simulink model "dx_hand_model"  (R2017b)
settings: Solver=ode3  StartTime=0.0  StopTime=inf  FixedStep=0.01  RelTol=1e-3  EnableMultiTasking=on
InitFcn:
  | cutFreq = 0.1; % T
  | sampleTime = 0.01;
  | filt = tf(1,[cutFreq 1]);
  | filt = c2d(filt,sampleTime);
  | 
  | cutFreq2 = 1;
  | filt2 = tf(1,[cutFreq2 1]);
  | filt2 = c2d(filt2,sampleTime);
  | 
  | cutFreq3 = 0.3;
  | filt3 = tf(1,[cutFreq3 1]);
  | filt3 = c2d(filt3,sampleTime);
  | 
  | update_param = 2;
  | 
  | ampliFactor = 1.60;
  | ampliFactorMiddle = 2.00;
  | ampliFactorDistal = 1;
  | 
  | % Set Hand Address
  | % RightHandAddress = '10.100.39.144';
  | RightHandAddress = '10.24.4.91';
  | Verosim = '10.100.39.22'
  | LeftHandAddress = '10.100.39.22'
  | 
  | max_force = 24; % Newton
model workspace (MAT data in the model file):
  SL_ROS_VariableLengthArrays_MaxSizes : struct (value not decoded)
libraries: robotlib x136, simulink_extras x27, simulink x16, etargetslib x2, dspnetwork x2
(part 3 of 19)

== system dx_hand_model/Get From Schunk/Get positions/Get Positions ==
  <Position> : Inport
  Data Type Conversion1 : DataTypeConversion  OutDataTypeStr=single
  Data Type Conversion2 : DataTypeConversion  OutDataTypeStr=single
  Demux : Demux  Outputs=9
  Display : Display
  Filter : Subsystem
  Filter1 : Subsystem
  Filter2 : Subsystem
  Filter3 : Subsystem
  Filter4 : Subsystem
  Filter5 : Subsystem
  Get Parameter3 : robotlib/Get Parameter  SourceLibraryInfo=This block requires Robotics System Toolbox  ParameterSource=Specify your own  ParameterName=/hand_exo/position/filt  ParameterType=double  ParameterMaxArrayLength=16  ParameterInitialValue=1.0  SampleTime=update_param  ShowErrorCodeOutput=on  ModelName=dx_hand_model  BlockId=ParamGet_dx_hand_model_3210
      settings: SourceProductName=Robotics System Toolbox  SourceProductBaseCode=RO
  Rate Transition : RateTransition
  Selector : Selector  IndexOptions=Index vector (dialog)  Indices=[1 2 3 4 5 6 7 8 9]  OutputSizes=1
  tag scope: act_IndexDistal=global, act_IndexProxi=global, act_MiddleDistal=global, act_MiddleProxi=global, act_Pinky=global, act_Ring=global
  wires:
  <Position>/1 -> Display/1, Selector/1
  Selector/1 -> Data Type Conversion2/1
  Demux/5 -> Filter2/2(in)
  Data Type Conversion2/1 -> Demux/1
  Demux/4 -> Filter1/2(in)
  Demux/6 -> Filter3/2(in)
  Filter1/1(out) -> [act_IndexProxi]
  Demux/3 -> Filter/2(in)
  Filter/1(out) -> [act_IndexDistal]
  Rate Transition/1 -> Data Type Conversion1/1
  Get Parameter3/1 -> Rate Transition/1
  Data Type Conversion1/1 -> Filter4/1(enable), Filter5/1(enable), Filter3/1(enable), Filter2/1(enable), Filter1/1(enable), Filter/1(enable)
  Filter2/1(out) -> [act_MiddleDistal]
  Filter3/1(out) -> [act_MiddleProxi]
  Filter5/1(out) -> [act_Ring]
  Demux/7 -> Filter5/2(in)
  Filter4/1(out) -> [act_Pinky]
  Demux/8 -> Filter4/2(in)

== system dx_hand_model/Index Finger/Force/Position Force Basic Architecture ==
  Display : Display
  Gain1 : Gain  Gain=1/360
  Maximum Torque : Gain  Gain=0.52
  Maximum Torque1 : Gain  Gain=0.04
  Mux : Mux  Inputs=2
  Normalize Current : Gain  Gain=1/688
  Sign : Gain  Gain=-1
  Sign1 : Gain
  pos_gains/dist : Subsystem
  pos_gains/prox : Subsystem
  force_vec : Outport
  wires:
  Mux/1 -> Display/1, force_vec/1
  pos_gains/dist/1(post_dist) -> Mux/2
  [CurrentIndexProximal] -> Normalize Current/1
  pos_gains/prox/1(post_prox) -> Mux/1
  [CurrentIndexDistal] -> Gain1/1
  Normalize Current/1 -> Maximum Torque/1
  Gain1/1 -> Maximum Torque1/1
  Maximum Torque/1 -> Sign/1
  Sign/1 -> pos_gains/prox/1(pre_prox)
  Maximum Torque1/1 -> Sign1/1
  Sign1/1 -> pos_gains/dist/1(pre_dist)

== system dx_hand_model/Index Finger/Force/Subsystem ==
  optim : Inport
  classic : Inport  Port=2
  Data Type Conversion1 : DataTypeConversion  OutDataTypeStr=single
  Get Parameter3 : robotlib/Get Parameter  SourceLibraryInfo=This block requires Robotics System Toolbox  ParameterSource=Specify your own  ParameterName=/hand_exo/index/modes/jacobian  ParameterType=double  ParameterMaxArrayLength=16  ParameterInitialValue=-1.0  SampleTime=update_param  ShowErrorCodeOutput=on  ModelName=dx_hand_model  BlockId=ParamGet_dx_hand_model_2644
      settings: SourceProductName=Robotics System Toolbox  SourceProductBaseCode=RO
  Rate Transition : RateTransition
  Switch : Switch  Criteria=u2 > Threshold
  J_out : Outport
  wires:
  Get Parameter3/1 -> Rate Transition/1
  Data Type Conversion1/1 -> Switch/2
  optim/1 -> Switch/1
  classic/1 -> Switch/3
  Switch/1 -> J_out/1
  Rate Transition/1 -> Data Type Conversion1/1

== system dx_hand_model/Index Finger/Pose Generator/Angular Potentiometer ==
  ADC : Inport
  Constant4 : Constant  Value=pi/2  OutDataTypeStr=single
  Data Type Conversion1 : DataTypeConversion  OutDataTypeStr=single
  Data Type Conversion2 : DataTypeConversion  OutDataTypeStr=double
  Display2 : Display
  Gain Aggiustato1 : Gain  Gain=330*pi/(1024*180)
  Get Parameter3 : robotlib/Get Parameter  SourceLibraryInfo=This block requires Robotics System Toolbox  ParameterSource=Specify your own  ParameterName=/hand_exo/index/calibration/set  ParameterType=double  ParameterMaxArrayLength=16  ParameterInitialValue=483  SampleTime=update_param  ShowErrorCodeOutput=on  ModelName=dx_hand_model  BlockId=ParamGet_dx_hand_model_2632
      settings: SourceProductName=Robotics System Toolbox  SourceProductBaseCode=RO
  Radians to Degrees1 : simulink_extras/Transformations/Radians to Degrees
  Rate Transition : RateTransition
  Set Parameter : robotlib/Set Parameter  SourceLibraryInfo=This block requires Robotics System Toolbox  ParameterSource=Specify your own  ParameterName=/hand_exo/index/calibration/get  ParameterType=double  ModelName=dx_hand_model  BlockId=ParamSet_dx_hand_model_2630
      settings: SourceProductName=Robotics System Toolbox  SourceProductBaseCode=RO
  Sum3 : Sum  Inputs=|+-
  Sum4 : Sum  Inputs=|+-
  Deg : Outport
  Rad : Outport  Port=2
  wires:
  Radians to Degrees1/1 -> Deg/1
  Sum4/1 -> Rad/1, Radians to Degrees1/1
  ADC/1 -> Data Type Conversion2/1, Sum3/1
  Sum3/1 -> Gain Aggiustato1/1
  Constant4/1 -> Sum4/1
  Gain Aggiustato1/1 -> Sum4/2
  Data Type Conversion2/1 -> Display2/1, Set Parameter/1
  Rate Transition/1 -> Data Type Conversion1/1
  Get Parameter3/1 -> Rate Transition/1
  Data Type Conversion1/1 -> Sum3/2

== system dx_hand_model/Index Finger/Pose Generator/Parameters ==
  In1 : Inport
  Data Type Conversion1 : DataTypeConversion  OutDataTypeStr=single
  Index Parameters : MATLAB Function  TreatAsAtomicUnit=on
  "to_dir_kin " : Outport
  wires:
  Index Parameters/1(y) -> Data Type Conversion1/1
  In1/1 -> Index Parameters/1(x)
  Data Type Conversion1/1 -> "to_dir_kin "/1

== system dx_hand_model/Index Finger/Pose Generator/Parametri Dito ==
  Get_from_ROS_param : Subsystem
  Hand Written : Subsystem
  Manual Switch : ManualSwitch
  Par : Outport
  wires:
  Get_from_ROS_param/1(param) -> Manual Switch/1
  Hand Written/1(param) -> Manual Switch/2
  Manual Switch/1 -> Par/1

== system dx_hand_model/Index Finger/Pose Generator/Record ==
  input : Inport
  param : Inport  Port=2
  output : Inport  Port=3
  Enable : EnablePort
  Mux2 : Mux  Inputs=3
  To Workspace : ToWorkspace  VariableName=index_pose  SampleTime=-1
  wires:
  Mux2/1 -> To Workspace/1
  param/1 -> Mux2/2
  output/1 -> Mux2/3
  input/1 -> Mux2/1

== system dx_hand_model/Index Finger/Pose Generator/Subsystem ==
  ADC : Inport
  Gain Aggiustato : Gain  Gain=50/1024
  "lx " : Outport
  wires:
  ADC/1 -> Gain Aggiustato/1
  Gain Aggiustato/1 -> "lx "/1

== system dx_hand_model/Index Finger/Position/Pre-Proc ==
  yes : Inport
  no : Inport  Port=2
  Data Type Conversion1 : DataTypeConversion  OutDataTypeStr=single
  Get Parameter3 : robotlib/Get Parameter  SourceLibraryInfo=This block requires Robotics System Toolbox  ParameterSource=Specify your own  ParameterName=/hand_exo/index/position/optim  ParameterType=double  ParameterMaxArrayLength=16  ParameterInitialValue=1.0  SampleTime=update_param  ShowErrorCodeOutput=on  ModelName=dx_hand_model  BlockId=ParamGet_dx_hand_model_3323
      settings: SourceProductName=Robotics System Toolbox  SourceProductBaseCode=RO
  Rate Transition : RateTransition
  Switch : Switch  Criteria=u2 > Threshold
  out : Outport
  wires:
  Get Parameter3/1 -> Rate Transition/1
  Rate Transition/1 -> Data Type Conversion1/1
  Data Type Conversion1/1 -> Switch/2
  yes/1 -> Switch/1
  no/1 -> Switch/3
  Switch/1 -> out/1

== system dx_hand_model/Index Finger/Position/active ==
  in : Inport
  Constant : Constant  Value=0  OutDataTypeStr=single
  Data Type Conversion1 : DataTypeConversion  OutDataTypeStr=single
  Get Parameter3 : robotlib/Get Parameter  SourceLibraryInfo=This block requires Robotics System Toolbox  ParameterSource=Specify your own  ParameterName=/hand_exo/index/position/proxi_d_act  ParameterType=double  ParameterMaxArrayLength=16  ParameterInitialValue=-1.0  SampleTime=update_param  ShowErrorCodeOutput=off  ModelName=dx_hand_model  BlockId=ParamGet_dx_hand_model_3464
      settings: SourceProductName=Robotics System Toolbox  SourceProductBaseCode=RO
  Rate Transition : RateTransition
  Switch : Switch  Criteria=u2 > Threshold
  out : Outport
  wires:
  Switch/1 -> out/1
  Data Type Conversion1/1 -> Switch/2
  Rate Transition/1 -> Data Type Conversion1/1
  Get Parameter3/1 -> Rate Transition/1
  in/1 -> Switch/1
  Constant/1 -> Switch/3

== system dx_hand_model/Index Finger/Position/active1 ==
  in : Inport
  Constant : Constant  Value=0  OutDataTypeStr=single
  Data Type Conversion1 : DataTypeConversion  OutDataTypeStr=single
  Get Parameter3 : robotlib/Get Parameter  SourceLibraryInfo=This block requires Robotics System Toolbox  ParameterSource=Specify your own  ParameterName=/hand_exo/index/position/dist_d_act  ParameterType=double  ParameterMaxArrayLength=16  ParameterInitialValue=-1.0  SampleTime=update_param  ShowErrorCodeOutput=off  ModelName=dx_hand_model  BlockId=ParamGet_dx_hand_model_3474
      settings: SourceProductName=Robotics System Toolbox  SourceProductBaseCode=RO
  Rate Transition : RateTransition
  Switch : Switch  Criteria=u2 > Threshold
  out : Outport
  wires:
  Switch/1 -> out/1
  Data Type Conversion1/1 -> Switch/2
  Rate Transition/1 -> Data Type Conversion1/1
  Get Parameter3/1 -> Rate Transition/1
  in/1 -> Switch/1
  Constant/1 -> Switch/3

== system dx_hand_model/Index Finger/Position/setGain ==
  in : Inport
  Data Type Conversion1 : DataTypeConversion  OutDataTypeStr=single
  Get Parameter3 : robotlib/Get Parameter  SourceLibraryInfo=This block requires Robotics System Toolbox  ParameterSource=Specify your own  ParameterName=/hand_exo/index/position/kp_p  ParameterType=double  ParameterMaxArrayLength=16  ParameterInitialValue=1.2  SampleTime=update_param  ShowErrorCodeOutput=off  ModelName=dx_hand_model  BlockId=ParamGet_dx_hand_model_3283
      settings: SourceProductName=Robotics System Toolbox  SourceProductBaseCode=RO
  Product : Product
  Rate Transition : RateTransition
  out : Outport
  wires:
  Product/1 -> out/1
  Data Type Conversion1/1 -> Product/1
  in/1 -> Product/2
  Rate Transition/1 -> Data Type Conversion1/1
  Get Parameter3/1 -> Rate Transition/1

== system dx_hand_model/Index Finger/Position/setGain  ==
  in : Inport
  Data Type Conversion1 : DataTypeConversion  OutDataTypeStr=single
  Get Parameter3 : robotlib/Get Parameter  SourceLibraryInfo=This block requires Robotics System Toolbox  ParameterSource=Specify your own  ParameterName=/hand_exo/index/position/kp_d  ParameterType=double  ParameterMaxArrayLength=16  ParameterInitialValue=0.2  SampleTime=update_param  ShowErrorCodeOutput=off  ModelName=dx_hand_model  BlockId=ParamGet_dx_hand_model_3296
      settings: SourceProductName=Robotics System Toolbox  SourceProductBaseCode=RO
  Product : Product
  Rate Transition : RateTransition
  out : Outport
  wires:
  Product/1 -> out/1
  Data Type Conversion1/1 -> Product/1
  in/1 -> Product/2
  Rate Transition/1 -> Data Type Conversion1/1
  Get Parameter3/1 -> Rate Transition/1

== system dx_hand_model/Index Finger/Position/setGain 1 ==
  in : Inport
  Data Type Conversion1 : DataTypeConversion  OutDataTypeStr=single
  Get Parameter3 : robotlib/Get Parameter  SourceLibraryInfo=This block requires Robotics System Toolbox  ParameterSource=Specify your own  ParameterName=/hand_exo/index/position/kd_p  ParameterType=double  ParameterMaxArrayLength=16  ParameterInitialValue=0.0  SampleTime=update_param  ShowErrorCodeOutput=off  ModelName=dx_hand_model  BlockId=ParamGet_dx_hand_model_3307
      settings: SourceProductName=Robotics System Toolbox  SourceProductBaseCode=RO
  Product : Product
  Rate Transition : RateTransition
  out : Outport
  wires:
  Product/1 -> out/1
  Data Type Conversion1/1 -> Product/1
  in/1 -> Product/2
  Rate Transition/1 -> Data Type Conversion1/1
  Get Parameter3/1 -> Rate Transition/1

== system dx_hand_model/Index Finger/Position/setGain 2 ==
  in : Inport
  Data Type Conversion1 : DataTypeConversion  OutDataTypeStr=single
  Get Parameter3 : robotlib/Get Parameter  SourceLibraryInfo=This block requires Robotics System Toolbox  ParameterSource=Specify your own  ParameterName=/hand_exo/index/position/kd_d  ParameterType=double  ParameterMaxArrayLength=16  ParameterInitialValue=0.0  SampleTime=update_param  ShowErrorCodeOutput=off  ModelName=dx_hand_model  BlockId=ParamGet_dx_hand_model_3314
      settings: SourceProductName=Robotics System Toolbox  SourceProductBaseCode=RO
  Product : Product
  Rate Transition : RateTransition
  out : Outport
  wires:
  Product/1 -> out/1
  Data Type Conversion1/1 -> Product/1
  in/1 -> Product/2
  Rate Transition/1 -> Data Type Conversion1/1
  Get Parameter3/1 -> Rate Transition/1

== system dx_hand_model/Index Finger/Send Position/setGain ==
  in : Inport
  Data Type Conversion1 : DataTypeConversion  OutDataTypeStr=single
  Get Parameter3 : robotlib/Get Parameter  SourceLibraryInfo=This block requires Robotics System Toolbox  ParameterSource=Specify your own  ParameterName=/hand_exo/index/schunk_gains/prox  ParameterType=double  ParameterMaxArrayLength=16  ParameterInitialValue=1.0  SampleTime=update_param  ShowErrorCodeOutput=off  ModelName=dx_hand_model  BlockId=ParamGet_dx_hand_model_3391
      settings: SourceProductName=Robotics System Toolbox  SourceProductBaseCode=RO
  Product : Product
  Rate Transition : RateTransition
  out : Outport
  wires:
  Product/1 -> out/1
  Data Type Conversion1/1 -> Product/1
  in/1 -> Product/2
  Rate Transition/1 -> Data Type Conversion1/1
  Get Parameter3/1 -> Rate Transition/1

== system dx_hand_model/Index Finger/Send Position/setGain1 ==
  in : Inport
  Data Type Conversion1 : DataTypeConversion  OutDataTypeStr=single
  Get Parameter3 : robotlib/Get Parameter  SourceLibraryInfo=This block requires Robotics System Toolbox  ParameterSource=Specify your own  ParameterName=/hand_exo/index/schunk_gains/dist  ParameterType=double  ParameterMaxArrayLength=16  ParameterInitialValue=1.0  SampleTime=update_param  ShowErrorCodeOutput=off  ModelName=dx_hand_model  BlockId=ParamGet_dx_hand_model_3398
      settings: SourceProductName=Robotics System Toolbox  SourceProductBaseCode=RO
  Product : Product
  Rate Transition : RateTransition
  out : Outport
  wires:
  Product/1 -> out/1
  Data Type Conversion1/1 -> Product/1
  in/1 -> Product/2
  Rate Transition/1 -> Data Type Conversion1/1
  Get Parameter3/1 -> Rate Transition/1

== system dx_hand_model/Middle Finger/Pose Generator/Angular Potentiometer ==
  ADC : Inport
  Constant : Constant  Value=pi/2  OutDataTypeStr=single
  Constant1 : Constant  Value=495  OutDataTypeStr=single
  Data Type Conversion1 : DataTypeConversion  OutDataTypeStr=single
  Data Type Conversion2 : DataTypeConversion  OutDataTypeStr=double
  Display : Display
  Display1 : Display
  Display2 : Display
  Gain Aggiustato : Gain  Gain=330*pi/(1024*180)
  Get Parameter3 : robotlib/Get Parameter  SourceLibraryInfo=This block requires Robotics System Toolbox  ParameterSource=Specify your own  ParameterName=/hand_exo/middle/calibration/set  ParameterType=double  ParameterMaxArrayLength=16  ParameterInitialValue=754  SampleTime=update_param  ShowErrorCodeOutput=on  ModelName=dx_hand_model  BlockId=ParamGet_dx_hand_model_2565
      settings: SourceProductName=Robotics System Toolbox  SourceProductBaseCode=RO
  Manual Switch : ManualSwitch
  Radians to Degrees : simulink_extras/Transformations/Radians to Degrees
  Rate Transition : RateTransition
  Set Parameter : robotlib/Set Parameter  SourceLibraryInfo=This block requires Robotics System Toolbox  ParameterSource=Specify your own  ParameterName=/hand_exo/middle/calibration/get  ParameterType=double  ModelName=dx_hand_model  BlockId=ParamSet_dx_hand_model_2567
      settings: SourceProductName=Robotics System Toolbox  SourceProductBaseCode=RO
  Sum1 : Sum  Inputs=|-+
  Sum2 : Sum  Inputs=|+-
  Deg : Outport
  Rad : Outport  Port=2
  wires:
  ADC/1 -> Data Type Conversion2/1, Sum2/1
  Radians to Degrees/1 -> Display1/1, Deg/1
  Gain Aggiustato/1 -> Display/1, Sum1/1
  Sum1/1 -> Radians to Degrees/1, Rad/1
  Constant/1 -> Sum1/2
  Sum2/1 -> Gain Aggiustato/1
  Get Parameter3/1 -> Rate Transition/1
  Data Type Conversion2/1 -> Set Parameter/1, Display2/1
  Rate Transition/1 -> Data Type Conversion1/1
  Data Type Conversion1/1 -> Manual Switch/1
  Manual Switch/1 -> Sum2/2
  Constant1/1 -> Manual Switch/2

== system dx_hand_model/Middle Finger/Pose Generator/Filtro ==
  pre : Inport
  Data Type Conversion1 : DataTypeConversion  OutDataTypeStr=single
  Data Type Conversion2 : DataTypeConversion  OutDataTypeStr=double
  Data Type Conversion3 : DataTypeConversion  OutDataTypeStr=double
  Filtro : MATLAB Function  TreatAsAtomicUnit=on
  Memory : Memory
  Memory1 : Memory
  post : Outport
  wires:
  Memory1/1 -> Data Type Conversion3/1
  Filtro/3(qo2) -> Memory1/1
  pre/1 -> Filtro/1(x)
  Filtro/2(qo1) -> Memory/1
  Memory/1 -> Data Type Conversion2/1
  Filtro/1(y) -> Data Type Conversion1/1
  Data Type Conversion1/1 -> post/1
  Data Type Conversion2/1 -> Filtro/2(qin1)
  Data Type Conversion3/1 -> Filtro/3(qin2)

== system dx_hand_model/Middle Finger/Pose Generator/Linear Potentiometer ==
  ADC : Inport
  Gain Aggiustato : Gain  Gain=50/1024
  mm : Outport
  wires:
  ADC/1 -> Gain Aggiustato/1
  Gain Aggiustato/1 -> mm/1

== system dx_hand_model/Middle Finger/Pose Generator/Parameters ==
  Par5 : Inport
  Data Type Conversion1 : DataTypeConversion  OutDataTypeStr=single
  Middle Parameters : MATLAB Function  TreatAsAtomicUnit=on
  to Direct Kin : Outport
  wires:
  Middle Parameters/1(y) -> Data Type Conversion1/1
  Data Type Conversion1/1 -> to Direct Kin/1
  Par5/1 -> Middle Parameters/1(x)

== system dx_hand_model/Middle Finger/Pose Generator/Parametri Dito ==
  Get_from_ROS_param : Subsystem
  Hand_written : Subsystem
  Manual Switch : ManualSwitch
  Par_5 : Outport
  wires:
  Hand_written/1(Out2) -> Manual Switch/2
  Get_from_ROS_param/1(param) -> Manual Switch/1
  Manual Switch/1 -> Par_5/1

== system dx_hand_model/Middle Finger/Pose Generator/Record ==
  input : Inport
  param : Inport  Port=2
  output : Inport  Port=3
  Enable : EnablePort
  Mux2 : Mux  Inputs=3
  To Workspace : ToWorkspace  VariableName=middle_pose  SampleTime=-1
  wires:
  Mux2/1 -> To Workspace/1
  param/1 -> Mux2/2
  input/1 -> Mux2/1
  output/1 -> Mux2/3

== system dx_hand_model/Middle Finger/Position-Force Architecture/Position Force Basic Architecture ==
  Display : Display
  Gain : Gain  Gain=1/680
  Gain1 : Gain  Gain=1/360
  Gain2 : Gain  Gain=0.52
  Gain3 : Gain  Gain=-1
  Gain4 : Gain  Gain=0.04
  Gain5 : Gain
  Mux : Mux  Inputs=2
  pos_gains/dist : Subsystem
  pos_gains/prox : Subsystem
  force_vec : Outport
  wires:
  Mux/1 -> Display/1, force_vec/1
  pos_gains/dist/1(post_dist) -> Mux/2
  [CurrentMiddleProximal] -> Gain/1
  pos_gains/prox/1(post_prox) -> Mux/1
  [CurrentMiddleDistal] -> Gain1/1
  Gain/1 -> Gain2/1
  Gain1/1 -> Gain4/1
  Gain2/1 -> Gain3/1
  Gain3/1 -> pos_gains/prox/1(pre_prox)
  Gain4/1 -> Gain5/1
  Gain5/1 -> pos_gains/dist/1(pre_dist)

== system dx_hand_model/Middle Finger/Position-Force Architecture/Subsystem ==
  optim : Inport
  classic : Inport  Port=2
  Data Type Conversion1 : DataTypeConversion  OutDataTypeStr=single
  Get Parameter3 : robotlib/Get Parameter  SourceLibraryInfo=This block requires Robotics System Toolbox  ParameterSource=Specify your own  ParameterName=/hand_exo/middle/modes/jacobian  ParameterType=double  ParameterMaxArrayLength=16  ParameterInitialValue=-1.0  SampleTime=update_param  ShowErrorCodeOutput=on  ModelName=dx_hand_model  BlockId=ParamGet_dx_hand_model_2571
      settings: SourceProductName=Robotics System Toolbox  SourceProductBaseCode=RO
  Rate Transition : RateTransition
  Switch : Switch  Criteria=u2 > Threshold
  J_out : Outport
  wires:
  Get Parameter3/1 -> Rate Transition/1
  Data Type Conversion1/1 -> Switch/2
  optim/1 -> Switch/1
  classic/1 -> Switch/3
  Switch/1 -> J_out/1
  Rate Transition/1 -> Data Type Conversion1/1

== system dx_hand_model/Middle Finger/Position-Position/Pre-Proc ==
  yes : Inport
  no : Inport  Port=2
  Data Type Conversion1 : DataTypeConversion  OutDataTypeStr=single
  Get Parameter3 : robotlib/Get Parameter  SourceLibraryInfo=This block requires Robotics System Toolbox  ParameterSource=Specify your own  ParameterName=/hand_exo/middle/position/optim  ParameterType=double  ParameterMaxArrayLength=16  ParameterInitialValue=1.0  SampleTime=update_param  ShowErrorCodeOutput=on  ModelName=dx_hand_model  BlockId=ParamGet_dx_hand_model_3348
      settings: SourceProductName=Robotics System Toolbox  SourceProductBaseCode=RO
  Rate Transition : RateTransition
  Switch : Switch  Criteria=u2 > Threshold
  out : Outport
  wires:
  Get Parameter3/1 -> Rate Transition/1
  Rate Transition/1 -> Data Type Conversion1/1
  Data Type Conversion1/1 -> Switch/2
  yes/1 -> Switch/1
  no/1 -> Switch/3
  Switch/1 -> out/1

== system dx_hand_model/Middle Finger/Position-Position/active ==
  in : Inport
  Constant : Constant  Value=0  OutDataTypeStr=single
  Data Type Conversion1 : DataTypeConversion  OutDataTypeStr=single
  Get Parameter3 : robotlib/Get Parameter  SourceLibraryInfo=This block requires Robotics System Toolbox  ParameterSource=Specify your own  ParameterName=/hand_exo/middle/position/proxi_d_act  ParameterType=double  ParameterMaxArrayLength=16  ParameterInitialValue=-1.0  SampleTime=update_param  ShowErrorCodeOutput=off  ModelName=dx_hand_model  BlockId=ParamGet_dx_hand_model_3482
      settings: SourceProductName=Robotics System Toolbox  SourceProductBaseCode=RO
  Rate Transition : RateTransition
  Switch : Switch  Criteria=u2 > Threshold
  out : Outport
  wires:
  Switch/1 -> out/1
  Data Type Conversion1/1 -> Switch/2
  Rate Transition/1 -> Data Type Conversion1/1
  Get Parameter3/1 -> Rate Transition/1
  in/1 -> Switch/1
  Constant/1 -> Switch/3

== system dx_hand_model/Middle Finger/Position-Position/active1 ==
  in : Inport
  Constant : Constant  Value=0  OutDataTypeStr=single
  Data Type Conversion1 : DataTypeConversion  OutDataTypeStr=single
  Get Parameter3 : robotlib/Get Parameter  SourceLibraryInfo=This block requires Robotics System Toolbox  ParameterSource=Specify your own  ParameterName=/hand_exo/middle/position/dist_d_act  ParameterType=double  ParameterMaxArrayLength=16  ParameterInitialValue=-1.0  SampleTime=update_param  ShowErrorCodeOutput=off  ModelName=dx_hand_model  BlockId=ParamGet_dx_hand_model_3490
      settings: SourceProductName=Robotics System Toolbox  SourceProductBaseCode=RO
  Rate Transition : RateTransition
  Switch : Switch  Criteria=u2 > Threshold
  out : Outport
  wires:
  Switch/1 -> out/1
  Data Type Conversion1/1 -> Switch/2
  Rate Transition/1 -> Data Type Conversion1/1
  Get Parameter3/1 -> Rate Transition/1
  in/1 -> Switch/1
  Constant/1 -> Switch/3

== system dx_hand_model/Middle Finger/Position-Position/setGain ==
  in : Inport
  Data Type Conversion1 : DataTypeConversion  OutDataTypeStr=single
  Get Parameter3 : robotlib/Get Parameter  SourceLibraryInfo=This block requires Robotics System Toolbox  ParameterSource=Specify your own  ParameterName=/hand_exo/middle/position/kp_p  ParameterType=double  ParameterMaxArrayLength=16  ParameterInitialValue=1.2  SampleTime=update_param  ShowErrorCodeOutput=off  ModelName=dx_hand_model  BlockId=ParamGet_dx_hand_model_3362
      settings: SourceProductName=Robotics System Toolbox  SourceProductBaseCode=RO
  Product : Product
  Rate Transition : RateTransition
  out : Outport
  wires:
  Product/1 -> out/1
  Data Type Conversion1/1 -> Product/1
  in/1 -> Product/2
  Rate Transition/1 -> Data Type Conversion1/1
  Get Parameter3/1 -> Rate Transition/1

== system dx_hand_model/Middle Finger/Position-Position/setGain  ==
  in : Inport
  Data Type Conversion1 : DataTypeConversion  OutDataTypeStr=single
  Get Parameter3 : robotlib/Get Parameter  SourceLibraryInfo=This block requires Robotics System Toolbox  ParameterSource=Specify your own  ParameterName=/hand_exo/middle/position/kp_d  ParameterType=double  ParameterMaxArrayLength=16  ParameterInitialValue=0.2  SampleTime=update_param  ShowErrorCodeOutput=off  ModelName=dx_hand_model  BlockId=ParamGet_dx_hand_model_3369
      settings: SourceProductName=Robotics System Toolbox  SourceProductBaseCode=RO
  Product : Product
  Rate Transition : RateTransition
  out : Outport
  wires:
  Product/1 -> out/1
  Data Type Conversion1/1 -> Product/1
  in/1 -> Product/2
  Rate Transition/1 -> Data Type Conversion1/1
  Get Parameter3/1 -> Rate Transition/1

== system dx_hand_model/Middle Finger/Position-Position/setGain 1 ==
  in : Inport
  Data Type Conversion1 : DataTypeConversion  OutDataTypeStr=single
  Get Parameter3 : robotlib/Get Parameter  SourceLibraryInfo=This block requires Robotics System Toolbox  ParameterSource=Specify your own  ParameterName=/hand_exo/middle/position/kd_p  ParameterType=double  ParameterMaxArrayLength=16  ParameterInitialValue=0.0  SampleTime=update_param  ShowErrorCodeOutput=off  ModelName=dx_hand_model  BlockId=ParamGet_dx_hand_model_3376
      settings: SourceProductName=Robotics System Toolbox  SourceProductBaseCode=RO
  Product : Product
  Rate Transition : RateTransition
  out : Outport
  wires:
  Product/1 -> out/1
  Data Type Conversion1/1 -> Product/1
  in/1 -> Product/2
  Rate Transition/1 -> Data Type Conversion1/1
  Get Parameter3/1 -> Rate Transition/1

== system dx_hand_model/Middle Finger/Position-Position/setGain 2 ==
  in : Inport
  Data Type Conversion1 : DataTypeConversion  OutDataTypeStr=single
  Get Parameter3 : robotlib/Get Parameter  SourceLibraryInfo=This block requires Robotics System Toolbox  ParameterSource=Specify your own  ParameterName=/hand_exo/middle/position/kd_d  ParameterType=double  ParameterMaxArrayLength=16  ParameterInitialValue=0.0  SampleTime=update_param  ShowErrorCodeOutput=off  ModelName=dx_hand_model  BlockId=ParamGet_dx_hand_model_3383
      settings: SourceProductName=Robotics System Toolbox  SourceProductBaseCode=RO
  Product : Product
  Rate Transition : RateTransition
  out : Outport
  wires:
  Product/1 -> out/1
  Data Type Conversion1/1 -> Product/1
  in/1 -> Product/2
  Rate Transition/1 -> Data Type Conversion1/1
  Get Parameter3/1 -> Rate Transition/1

== system dx_hand_model/Pinky Finger/Pose Generator/Angular Potentiometer ==
  ADC : Inport
  Constant : Constant  Value=pi/2  OutDataTypeStr=single
  Constant1 : Constant  Value=495  OutDataTypeStr=single
  Data Type Conversion1 : DataTypeConversion  OutDataTypeStr=single
  Data Type Conversion2 : DataTypeConversion  OutDataTypeStr=double
  Display : Display
  Display1 : Display
  Display2 : Display
  Gain Aggiustato : Gain  Gain=330*pi/(1024*180)
  Get Parameter3 : robotlib/Get Parameter  SourceLibraryInfo=This block requires Robotics System Toolbox  ParameterSource=Specify your own  ParameterName=/hand_exo/pinky/calibration/set  ParameterType=double  ParameterMaxArrayLength=16  ParameterInitialValue=754  SampleTime=update_param  ShowErrorCodeOutput=on  ModelName=dx_hand_model  BlockId=ParamGet_dx_hand_model_4616
      settings: SourceProductName=Robotics System Toolbox  SourceProductBaseCode=RO
  Manual Switch : ManualSwitch
  Radians to Degrees : simulink_extras/Transformations/Radians to Degrees
  Rate Transition : RateTransition
  Set Parameter : robotlib/Set Parameter  SourceLibraryInfo=This block requires Robotics System Toolbox  ParameterSource=Specify your own  ParameterName=/hand_exo/pinky/calibration/get  ParameterType=double  ModelName=dx_hand_model  BlockId=ParamSet_dx_hand_model_4620
      settings: SourceProductName=Robotics System Toolbox  SourceProductBaseCode=RO
  Sum1 : Sum  Inputs=|-+
  Sum2 : Sum  Inputs=|+-
  Deg : Outport
  Rad : Outport  Port=2
  wires:
  ADC/1 -> Data Type Conversion2/1, Sum2/1
  Radians to Degrees/1 -> Display1/1, Deg/1
  Gain Aggiustato/1 -> Display/1, Sum1/1
  Sum1/1 -> Radians to Degrees/1, Rad/1
  Constant/1 -> Sum1/2
  Sum2/1 -> Gain Aggiustato/1
  Get Parameter3/1 -> Rate Transition/1
  Data Type Conversion2/1 -> Set Parameter/1, Display2/1
  Rate Transition/1 -> Data Type Conversion1/1
  Data Type Conversion1/1 -> Manual Switch/1
  Manual Switch/1 -> Sum2/2
  Constant1/1 -> Manual Switch/2

== system dx_hand_model/Pinky Finger/Pose Generator/Linear Potentiometer ==
  ADC : Inport
  Gain Aggiustato : Gain  Gain=50/1024
  mm : Outport
  wires:
  ADC/1 -> Gain Aggiustato/1
  Gain Aggiustato/1 -> mm/1

== system dx_hand_model/Pinky Finger/Pose Generator/Parametri Ring ==
  Get_from_ROS_param : Subsystem
  Hand_written : Subsystem
  Manual Switch : ManualSwitch
  Par_5 : Outport
  wires:
  Hand_written/1(Out2) -> Manual Switch/2
  Get_from_ROS_param/1(param) -> Manual Switch/1
  Manual Switch/1 -> Par_5/1

== system dx_hand_model/Pinky Finger/Pose Generator/Pinky Parameters ==
  Par5 : Inport
  Data Type Conversion1 : DataTypeConversion  OutDataTypeStr=single
  Pinky Parameters : MATLAB Function  TreatAsAtomicUnit=on
  to Direct Kin : Outport
  wires:
  Pinky Parameters/1(y) -> Data Type Conversion1/1
  Data Type Conversion1/1 -> to Direct Kin/1
  Par5/1 -> Pinky Parameters/1(x)

== system dx_hand_model/Pinky Finger/Pose Generator/Record ==
  input : Inport
  param : Inport  Port=2
  output : Inport  Port=3
  Enable : EnablePort
  Mux2 : Mux  Inputs=3
  To Workspace : ToWorkspace  VariableName=pinky_pose  SampleTime=-1
  wires:
  Mux2/1 -> To Workspace/1
  param/1 -> Mux2/2
  input/1 -> Mux2/1
  output/1 -> Mux2/3

== system dx_hand_model/Pinky Finger/Position-Force Architecture/Position Force Basic Architecture ==
  Display : Display
  Gain1 : Gain  Gain=1/360
  Gain2 : Gain
  Gain3 : Gain  Gain=0.03
  Mux : Mux  Inputs=2
  f_gains/dist : Subsystem
  f_gains/prox : Subsystem
  force_vec : Outport
  wires:
  Mux/1 -> Display/1, force_vec/1
  f_gains/dist/1(post_dist) -> Mux/2
  [CurrentPinky] -> Gain1/1
  f_gains/prox/1(post_prox) -> Mux/1
  Gain1/1 -> Gain3/1
  Gain2/1 -> f_gains/dist/1(pre_dist), f_gains/prox/1(pre_prox)
  Gain3/1 -> Gain2/1

== system dx_hand_model/Pinky Finger/Position-Force Architecture/Subsystem ==
  optim : Inport
  classic : Inport  Port=2
  Data Type Conversion1 : DataTypeConversion  OutDataTypeStr=single
  Get Parameter3 : robotlib/Get Parameter  SourceLibraryInfo=This block requires Robotics System Toolbox  ParameterSource=Specify your own  ParameterName=/hand_exo/pinky/modes/jacobian  ParameterType=double  ParameterMaxArrayLength=16  ParameterInitialValue=-1.0  SampleTime=update_param  ShowErrorCodeOutput=on  ModelName=dx_hand_model  BlockId=ParamGet_dx_hand_model_4720
      settings: SourceProductName=Robotics System Toolbox  SourceProductBaseCode=RO
  Rate Transition : RateTransition
  Switch : Switch  Criteria=u2 > Threshold
  J_out : Outport
  wires:
  Get Parameter3/1 -> Rate Transition/1
  Data Type Conversion1/1 -> Switch/2
  optim/1 -> Switch/1
  classic/1 -> Switch/3
  Switch/1 -> J_out/1
  Rate Transition/1 -> Data Type Conversion1/1

== system dx_hand_model/Pinky Finger/Position-Position/Pre-Proc ==
  yes : Inport
  no : Inport  Port=2
  Data Type Conversion1 : DataTypeConversion  OutDataTypeStr=single
  Get Parameter3 : robotlib/Get Parameter  SourceLibraryInfo=This block requires Robotics System Toolbox  ParameterSource=Specify your own  ParameterName=/hand_exo/pinky/position/optim  ParameterType=double  ParameterMaxArrayLength=16  ParameterInitialValue=1.0  SampleTime=update_param  ShowErrorCodeOutput=on  ModelName=dx_hand_model  BlockId=ParamGet_dx_hand_model_4743
      settings: SourceProductName=Robotics System Toolbox  SourceProductBaseCode=RO
  Rate Transition : RateTransition
  Switch : Switch  Criteria=u2 > Threshold
  out : Outport
  wires:
  Get Parameter3/1 -> Rate Transition/1
  Rate Transition/1 -> Data Type Conversion1/1
  Data Type Conversion1/1 -> Switch/2
  yes/1 -> Switch/1
  no/1 -> Switch/3
  Switch/1 -> out/1

== system dx_hand_model/Pinky Finger/Position-Position/active ==
  in : Inport
  Constant : Constant  Value=0  OutDataTypeStr=single
  Data Type Conversion1 : DataTypeConversion  OutDataTypeStr=single
  Get Parameter3 : robotlib/Get Parameter  SourceLibraryInfo=This block requires Robotics System Toolbox  ParameterSource=Specify your own  ParameterName=/hand_exo/pinky/position/proxi_d_act  ParameterType=double  ParameterMaxArrayLength=16  ParameterInitialValue=-1.0  SampleTime=update_param  ShowErrorCodeOutput=off  ModelName=dx_hand_model  BlockId=ParamGet_dx_hand_model_4758
      settings: SourceProductName=Robotics System Toolbox  SourceProductBaseCode=RO
  Rate Transition : RateTransition
  Switch : Switch  Criteria=u2 > Threshold
  out : Outport
  wires:
  Switch/1 -> out/1
  Data Type Conversion1/1 -> Switch/2
  Rate Transition/1 -> Data Type Conversion1/1
  Get Parameter3/1 -> Rate Transition/1
  in/1 -> Switch/1
  Constant/1 -> Switch/3

== system dx_hand_model/Pinky Finger/Position-Position/active1 ==
  in : Inport
  Constant : Constant  Value=0  OutDataTypeStr=single
  Data Type Conversion1 : DataTypeConversion  OutDataTypeStr=single
  Get Parameter3 : robotlib/Get Parameter  SourceLibraryInfo=This block requires Robotics System Toolbox  ParameterSource=Specify your own  ParameterName=/hand_exo/pinky/position/dist_d_act  ParameterType=double  ParameterMaxArrayLength=16  ParameterInitialValue=-1.0  SampleTime=update_param  ShowErrorCodeOutput=off  ModelName=dx_hand_model  BlockId=ParamGet_dx_hand_model_4766
      settings: SourceProductName=Robotics System Toolbox  SourceProductBaseCode=RO
  Rate Transition : RateTransition
  Switch : Switch  Criteria=u2 > Threshold
  out : Outport
  wires:
  Switch/1 -> out/1
  Data Type Conversion1/1 -> Switch/2
  Rate Transition/1 -> Data Type Conversion1/1
  Get Parameter3/1 -> Rate Transition/1
  in/1 -> Switch/1
  Constant/1 -> Switch/3

== system dx_hand_model/Pinky Finger/Position-Position/setGain ==
  in : Inport
  Data Type Conversion1 : DataTypeConversion  OutDataTypeStr=single
  Get Parameter3 : robotlib/Get Parameter  SourceLibraryInfo=This block requires Robotics System Toolbox  ParameterSource=Specify your own  ParameterName=/hand_exo/pinky/position/kp_p  ParameterType=double  ParameterMaxArrayLength=16  ParameterInitialValue=1.2  SampleTime=update_param  ShowErrorCodeOutput=off  ModelName=dx_hand_model  BlockId=ParamGet_dx_hand_model_4773
      settings: SourceProductName=Robotics System Toolbox  SourceProductBaseCode=RO
  Product : Product
  Rate Transition : RateTransition
  out : Outport
  wires:
  Product/1 -> out/1
  Data Type Conversion1/1 -> Product/1
  in/1 -> Product/2
  Rate Transition/1 -> Data Type Conversion1/1
  Get Parameter3/1 -> Rate Transition/1

== system dx_hand_model/Pinky Finger/Position-Position/setGain  ==
  in : Inport
  Data Type Conversion1 : DataTypeConversion  OutDataTypeStr=single
  Get Parameter3 : robotlib/Get Parameter  SourceLibraryInfo=This block requires Robotics System Toolbox  ParameterSource=Specify your own  ParameterName=/hand_exo/pinky/position/kp_d  ParameterType=double  ParameterMaxArrayLength=16  ParameterInitialValue=0.2  SampleTime=update_param  ShowErrorCodeOutput=off  ModelName=dx_hand_model  BlockId=ParamGet_dx_hand_model_4780
      settings: SourceProductName=Robotics System Toolbox  SourceProductBaseCode=RO
  Product : Product
  Rate Transition : RateTransition
  out : Outport
  wires:
  Product/1 -> out/1
  Data Type Conversion1/1 -> Product/1
  in/1 -> Product/2
  Rate Transition/1 -> Data Type Conversion1/1
  Get Parameter3/1 -> Rate Transition/1

== system dx_hand_model/Pinky Finger/Position-Position/setGain 1 ==
  in : Inport
  Data Type Conversion1 : DataTypeConversion  OutDataTypeStr=single
  Get Parameter3 : robotlib/Get Parameter  SourceLibraryInfo=This block requires Robotics System Toolbox  ParameterSource=Specify your own  ParameterName=/hand_exo/pinky/position/kd_p  ParameterType=double  ParameterMaxArrayLength=16  ParameterInitialValue=0.0  SampleTime=update_param  ShowErrorCodeOutput=off  ModelName=dx_hand_model  BlockId=ParamGet_dx_hand_model_4787
      settings: SourceProductName=Robotics System Toolbox  SourceProductBaseCode=RO
  Product : Product
  Rate Transition : RateTransition
  out : Outport
  wires:
  Product/1 -> out/1
  Data Type Conversion1/1 -> Product/1
  in/1 -> Product/2
  Rate Transition/1 -> Data Type Conversion1/1
  Get Parameter3/1 -> Rate Transition/1

== system dx_hand_model/Pinky Finger/Position-Position/setGain 2 ==
  in : Inport
  Data Type Conversion1 : DataTypeConversion  OutDataTypeStr=single
  Get Parameter3 : robotlib/Get Parameter  SourceLibraryInfo=This block requires Robotics System Toolbox  ParameterSource=Specify your own  ParameterName=/hand_exo/pinky/position/kd_d  ParameterType=double  ParameterMaxArrayLength=16  ParameterInitialValue=0.0  SampleTime=update_param  ShowErrorCodeOutput=off  ModelName=dx_hand_model  BlockId=ParamGet_dx_hand_model_4794
      settings: SourceProductName=Robotics System Toolbox  SourceProductBaseCode=RO
  Product : Product
  Rate Transition : RateTransition
  out : Outport
  wires:
  Product/1 -> out/1
  Data Type Conversion1/1 -> Product/1
  in/1 -> Product/2
  Rate Transition/1 -> Data Type Conversion1/1
  Get Parameter3/1 -> Rate Transition/1

== system dx_hand_model/Ring Finger /Pose Generator/Angular Potentiometer ==
  ADC : Inport
  Constant : Constant  Value=pi/2  OutDataTypeStr=single
  Constant1 : Constant  Value=495  OutDataTypeStr=single
  Data Type Conversion1 : DataTypeConversion  OutDataTypeStr=single
  Data Type Conversion2 : DataTypeConversion  OutDataTypeStr=double
  Display : Display
  Display1 : Display
  Display2 : Display
  Gain Aggiustato : Gain  Gain=330*pi/(1024*180)
  Get Parameter3 : robotlib/Get Parameter  SourceLibraryInfo=This block requires Robotics System Toolbox  ParameterSource=Specify your own  ParameterName=/hand_exo/ring/calibration/set  ParameterType=double  ParameterMaxArrayLength=16  ParameterInitialValue=754  SampleTime=update_param  ShowErrorCodeOutput=on  ModelName=dx_hand_model  BlockId=ParamGet_dx_hand_model_4319
      settings: SourceProductName=Robotics System Toolbox  SourceProductBaseCode=RO
  Manual Switch : ManualSwitch
  Radians to Degrees : simulink_extras/Transformations/Radians to Degrees
  Rate Transition : RateTransition
  Set Parameter : robotlib/Set Parameter  SourceLibraryInfo=This block requires Robotics System Toolbox  ParameterSource=Specify your own  ParameterName=/hand_exo/ring/calibration/get  ParameterType=double  ModelName=dx_hand_model  BlockId=ParamSet_dx_hand_model_4323
      settings: SourceProductName=Robotics System Toolbox  SourceProductBaseCode=RO
  Sum1 : Sum  Inputs=|-+
  Sum2 : Sum  Inputs=|+-
  Deg : Outport
  Rad : Outport  Port=2
  wires:
  ADC/1 -> Data Type Conversion2/1, Sum2/1
  Radians to Degrees/1 -> Display1/1, Deg/1
  Gain Aggiustato/1 -> Display/1, Sum1/1
  Sum1/1 -> Radians to Degrees/1, Rad/1
  Constant/1 -> Sum1/2
  Sum2/1 -> Gain Aggiustato/1
  Get Parameter3/1 -> Rate Transition/1
  Data Type Conversion2/1 -> Set Parameter/1, Display2/1
  Rate Transition/1 -> Data Type Conversion1/1
  Data Type Conversion1/1 -> Manual Switch/1
  Manual Switch/1 -> Sum2/2
  Constant1/1 -> Manual Switch/2

== system dx_hand_model/Ring Finger /Pose Generator/Linear Potentiometer ==
  ADC : Inport
  Gain Aggiustato : Gain  Gain=50/1024
  mm : Outport
  wires:
  ADC/1 -> Gain Aggiustato/1
  Gain Aggiustato/1 -> mm/1

== system dx_hand_model/Ring Finger /Pose Generator/Parametri Ring ==
  Get_from_ROS_param : Subsystem
  Hand_written : Subsystem
  Manual Switch : ManualSwitch
  Par_5 : Outport
  wires:
  Hand_written/1(Out2) -> Manual Switch/2
  Get_from_ROS_param/1(param) -> Manual Switch/1
  Manual Switch/1 -> Par_5/1

== system dx_hand_model/Ring Finger /Pose Generator/Record ==
  input : Inport
  param : Inport  Port=2
  output : Inport  Port=3
  Enable : EnablePort
  Mux2 : Mux  Inputs=3
  To Workspace : ToWorkspace  VariableName=ring_pose  SampleTime=-1
  wires:
  Mux2/1 -> To Workspace/1
  param/1 -> Mux2/2
  input/1 -> Mux2/1
  output/1 -> Mux2/3

== system dx_hand_model/Ring Finger /Pose Generator/Ring Parameters ==
  Par5 : Inport
  Data Type Conversion1 : DataTypeConversion  OutDataTypeStr=single
  Ring Parameters : MATLAB Function  TreatAsAtomicUnit=on
  to Direct Kin : Outport
  wires:
  Ring Parameters/1(y) -> Data Type Conversion1/1
  Data Type Conversion1/1 -> to Direct Kin/1
  Par5/1 -> Ring Parameters/1(x)

== system dx_hand_model/Ring Finger /Position-Force Architecture/Position Force Basic Architecture ==
  Display : Display
  Gain1 : Gain  Gain=1/360
  Gain2 : Gain
  Gain3 : Gain  Gain=0.06
  Mux : Mux  Inputs=2
  pos_gains/dist : Subsystem
  pos_gains/prox : Subsystem
  force_vec : Outport
  wires:
  Mux/1 -> Display/1, force_vec/1
  pos_gains/dist/1(post_dist) -> Mux/2
  [CurrentRing] -> Gain1/1
  pos_gains/prox/1(post_prox) -> Mux/1
  Gain1/1 -> Gain3/1
  Gain2/1 -> pos_gains/dist/1(pre_dist), pos_gains/prox/1(pre_prox)
  Gain3/1 -> Gain2/1

== system dx_hand_model/Ring Finger /Position-Force Architecture/Subsystem ==
  optim : Inport
  classic : Inport  Port=2
  Data Type Conversion1 : DataTypeConversion  OutDataTypeStr=single
  Get Parameter3 : robotlib/Get Parameter  SourceLibraryInfo=This block requires Robotics System Toolbox  ParameterSource=Specify your own  ParameterName=/hand_exo/ring/modes/jacobian  ParameterType=double  ParameterMaxArrayLength=16  ParameterInitialValue=-1.0  SampleTime=update_param  ShowErrorCodeOutput=on  ModelName=dx_hand_model  BlockId=ParamGet_dx_hand_model_4434
      settings: SourceProductName=Robotics System Toolbox  SourceProductBaseCode=RO
  Rate Transition : RateTransition
  Switch : Switch  Criteria=u2 > Threshold
  J_out : Outport
  wires:
  Get Parameter3/1 -> Rate Transition/1
  Data Type Conversion1/1 -> Switch/2
  optim/1 -> Switch/1
  classic/1 -> Switch/3
  Switch/1 -> J_out/1
  Rate Transition/1 -> Data Type Conversion1/1

== system dx_hand_model/Ring Finger /Position-Position/Pre-Proc ==
  yes : Inport
  no : Inport  Port=2
  Data Type Conversion1 : DataTypeConversion  OutDataTypeStr=single
  Get Parameter3 : robotlib/Get Parameter  SourceLibraryInfo=This block requires Robotics System Toolbox  ParameterSource=Specify your own  ParameterName=/hand_exo/ring/position/optim  ParameterType=double  ParameterMaxArrayLength=16  ParameterInitialValue=1.0  SampleTime=update_param  ShowErrorCodeOutput=on  ModelName=dx_hand_model  BlockId=ParamGet_dx_hand_model_4457
      settings: SourceProductName=Robotics System Toolbox  SourceProductBaseCode=RO
  Rate Transition : RateTransition
  Switch : Switch  Criteria=u2 > Threshold
  out : Outport
  wires:
  Get Parameter3/1 -> Rate Transition/1
  Rate Transition/1 -> Data Type Conversion1/1
  Data Type Conversion1/1 -> Switch/2
  yes/1 -> Switch/1
  no/1 -> Switch/3
  Switch/1 -> out/1

== system dx_hand_model/Ring Finger /Position-Position/active ==
  in : Inport
  Constant : Constant  Value=0  OutDataTypeStr=single
  Data Type Conversion1 : DataTypeConversion  OutDataTypeStr=single
  Get Parameter3 : robotlib/Get Parameter  SourceLibraryInfo=This block requires Robotics System Toolbox  ParameterSource=Specify your own  ParameterName=/hand_exo/ring/position/proxi_d_act  ParameterType=double  ParameterMaxArrayLength=16  ParameterInitialValue=-1.0  SampleTime=update_param  ShowErrorCodeOutput=off  ModelName=dx_hand_model  BlockId=ParamGet_dx_hand_model_4472
      settings: SourceProductName=Robotics System Toolbox  SourceProductBaseCode=RO
  Rate Transition : RateTransition
  Switch : Switch  Criteria=u2 > Threshold
  out : Outport
  wires:
  Switch/1 -> out/1
  Data Type Conversion1/1 -> Switch/2
  Rate Transition/1 -> Data Type Conversion1/1
  Get Parameter3/1 -> Rate Transition/1
  in/1 -> Switch/1
  Constant/1 -> Switch/3

== system dx_hand_model/Ring Finger /Position-Position/active1 ==
  in : Inport
  Constant : Constant  Value=0  OutDataTypeStr=single
  Data Type Conversion1 : DataTypeConversion  OutDataTypeStr=single
  Get Parameter3 : robotlib/Get Parameter  SourceLibraryInfo=This block requires Robotics System Toolbox  ParameterSource=Specify your own  ParameterName=/hand_exo/ring/position/dist_d_act  ParameterType=double  ParameterMaxArrayLength=16  ParameterInitialValue=-1.0  SampleTime=update_param  ShowErrorCodeOutput=off  ModelName=dx_hand_model  BlockId=ParamGet_dx_hand_model_4480
      settings: SourceProductName=Robotics System Toolbox  SourceProductBaseCode=RO
  Rate Transition : RateTransition
  Switch : Switch  Criteria=u2 > Threshold
  out : Outport
  wires:
  Switch/1 -> out/1
  Data Type Conversion1/1 -> Switch/2
  Rate Transition/1 -> Data Type Conversion1/1
  Get Parameter3/1 -> Rate Transition/1
  in/1 -> Switch/1
  Constant/1 -> Switch/3

== system dx_hand_model/Ring Finger /Position-Position/setGain ==
  in : Inport
  Data Type Conversion1 : DataTypeConversion  OutDataTypeStr=single
  Get Parameter3 : robotlib/Get Parameter  SourceLibraryInfo=This block requires Robotics System Toolbox  ParameterSource=Specify your own  ParameterName=/hand_exo/ring/position/kp_p  ParameterType=double  ParameterMaxArrayLength=16  ParameterInitialValue=1.2  SampleTime=update_param  ShowErrorCodeOutput=off  ModelName=dx_hand_model  BlockId=ParamGet_dx_hand_model_4487
      settings: SourceProductName=Robotics System Toolbox  SourceProductBaseCode=RO
  Product : Product
  Rate Transition : RateTransition
  out : Outport
  wires:
  Product/1 -> out/1
  Data Type Conversion1/1 -> Product/1
  in/1 -> Product/2
  Rate Transition/1 -> Data Type Conversion1/1
  Get Parameter3/1 -> Rate Transition/1

== system dx_hand_model/Ring Finger /Position-Position/setGain  ==
  in : Inport
  Data Type Conversion1 : DataTypeConversion  OutDataTypeStr=single
  Get Parameter3 : robotlib/Get Parameter  SourceLibraryInfo=This block requires Robotics System Toolbox  ParameterSource=Specify your own  ParameterName=/hand_exo/ring/position/kp_d  ParameterType=double  ParameterMaxArrayLength=16  ParameterInitialValue=0.2  SampleTime=update_param  ShowErrorCodeOutput=off  ModelName=dx_hand_model  BlockId=ParamGet_dx_hand_model_4494
      settings: SourceProductName=Robotics System Toolbox  SourceProductBaseCode=RO
  Product : Product
  Rate Transition : RateTransition
  out : Outport
  wires:
  Product/1 -> out/1
  Data Type Conversion1/1 -> Product/1
  in/1 -> Product/2
  Rate Transition/1 -> Data Type Conversion1/1
  Get Parameter3/1 -> Rate Transition/1

== system dx_hand_model/Ring Finger /Position-Position/setGain 1 ==
  in : Inport
  Data Type Conversion1 : DataTypeConversion  OutDataTypeStr=single
  Get Parameter3 : robotlib/Get Parameter  SourceLibraryInfo=This block requires Robotics System Toolbox  ParameterSource=Specify your own  ParameterName=/hand_exo/ring/position/kd_p  ParameterType=double  ParameterMaxArrayLength=16  ParameterInitialValue=0.0  SampleTime=update_param  ShowErrorCodeOutput=off  ModelName=dx_hand_model  BlockId=ParamGet_dx_hand_model_4501
      settings: SourceProductName=Robotics System Toolbox  SourceProductBaseCode=RO
  Product : Product
  Rate Transition : RateTransition
  out : Outport
  wires:
  Product/1 -> out/1
  Data Type Conversion1/1 -> Product/1
  in/1 -> Product/2
  Rate Transition/1 -> Data Type Conversion1/1
  Get Parameter3/1 -> Rate Transition/1

== system dx_hand_model/Ring Finger /Position-Position/setGain 2 ==
  in : Inport
  Data Type Conversion1 : DataTypeConversion  OutDataTypeStr=single
  Get Parameter3 : robotlib/Get Parameter  SourceLibraryInfo=This block requires Robotics System Toolbox  ParameterSource=Specify your own  ParameterName=/hand_exo/ring/position/kd_d  ParameterType=double  ParameterMaxArrayLength=16  ParameterInitialValue=0.0  SampleTime=update_param  ShowErrorCodeOutput=off  ModelName=dx_hand_model  BlockId=ParamGet_dx_hand_model_4508
      settings: SourceProductName=Robotics System Toolbox  SourceProductBaseCode=RO
  Product : Product
  Rate Transition : RateTransition
  out : Outport
  wires:
  Product/1 -> out/1
  Data Type Conversion1/1 -> Product/1
  in/1 -> Product/2
  Rate Transition/1 -> Data Type Conversion1/1
  Get Parameter3/1 -> Rate Transition/1

== system dx_hand_model/Send to Schunk/Send data to Ros/zzz3 ==
